simulink model "PhantomX_MK4"  (R2023a)
settings: Solver=FixedStepAuto  StartTime=0.0  StopTime=inf  FixedStep=0.00005  RelTol=1e-3
values from neighbouring files (symbols this model uses):
  angle_offsets_LF_RB = [45, 14.03624347, 60.58440117]    [InitialisationScript.m]    (also in simulation_setup.m)
  angle_offsets_middle = [0, 14.03624347, 60.58440117]    [InitialisationScript.m]    (also in simulation_setup.m)
  angle_offsets_RF_LB = [-45, 14.03624347, 60.58440117]    [InitialisationScript.m]    (also in simulation_setup.m)
  N = 16    [rl_setup.m]
  pid_D = 1    [InitialisationScript.m]    (also in simulation_setup.m)
  pid_filter_N = 100    [InitialisationScript.m]    (also in simulation_setup.m = 1000)
  pid_I = 0.2    [InitialisationScript.m]    (also in simulation_setup.m = 0.1)
  pid_P = 3    [InitialisationScript.m]    (also in simulation_setup.m = 600)
  x_offset = 0.2    [InitialisationScript.m]
  z_offset = -0.14    [InitialisationScript.m]
undefined symbols (not defined in the file or in its folder): LBL_sensory_data, left_side_torques, LFL_sensory_data, LML_sensory_data, RBL_sensory_data, RFL_sensory_data, right_side_torques, RML_sensory_data, X, Y, Z
libraries: sm_lib x30, slpidlib x18, Custom_Library x13, robotmaniplib x6, nesl_utility x3, rllib x1, simulink_extras x1
(part 4 of 4)

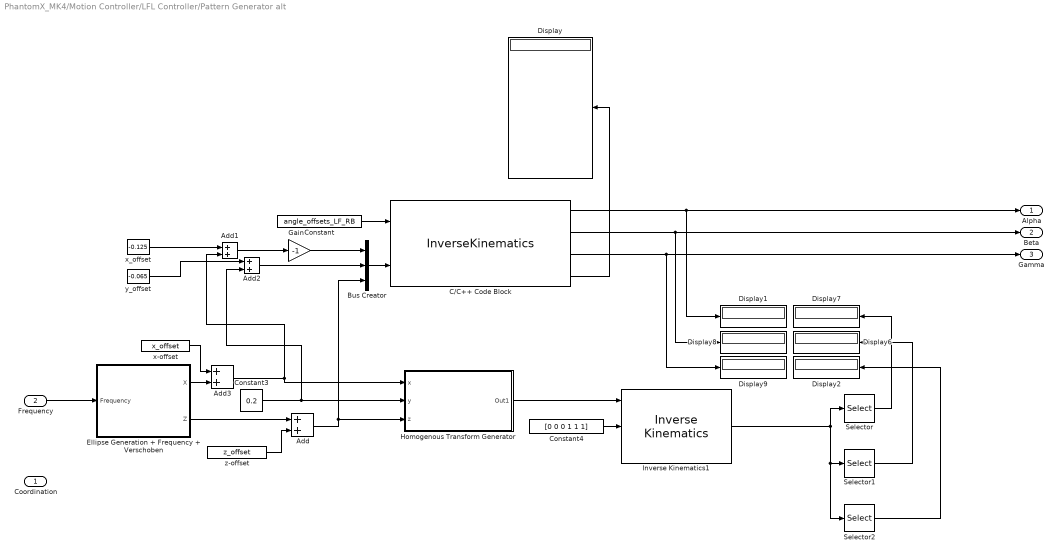
== system PhantomX_MK4/Motion Controller/LFL Controller/Pattern Generator alt ==
  Coordination : Inport
  Frequency : Inport  Port=2
  Add{,1..3} (4 alike) : Sum
  Bus Creator : BusCreator  Inputs=3
  C/C++ Code Block : S-Function  FunctionName=InverseKinematics  SFunctionModules=InverseKinematics_wrapper.c  SFunctionDeploymentMode=off  EnableBusSupport=off  mask(S-Function Builder){}
      mask help: Simulink:masks:SFunctionBuilder_MD
      mask init: same as PhantomX_MK4/Motion Controller/LBL Controller/Pattern Generator alt/C/C++ Code Block
      settings: CopyFcn=set_param(gcbh,'LinkStatus','none')  OpenFcn=sfunctionwizard(gcbh)
      mask Display:
      | plot(val(:,1),val(:,2))
      | disp(sys)
      | port_label('input',1,'angle_offsets')
      | port_label('input',2,'coordinates')
      | port_label('output',1,'alpha')
      | port_label('output',2,'beta')
      | port_label('output',3,'gamma')
      | port_label('output',4,'debug')
  Constant : Constant  Value=angle_offsets_LF_RB
  Constant3 : Constant  Value=0.2
  Constant4 : Constant  Value=[0 0 0 1 1 1]
  Display{,1..2,6..9} (7 alike) : Display
  Ellipse Generation + Frequency + Verschoben : Subsystem
  Gain : Gain  Gain=-1
  Homogenous Transform Generator : Subsystem
  Inverse Kinematics1 : robotmaniplib/Inverse Kinematics  RigidBodyTree=phantomX_mk4  EndEffector=PhantomX_MK4/left_front_foot_link  ShowInfo=off  SolverName=BFGS Gradient Projection  EnforceJointLimits=on  MaxIterations=30  MaxTime=0.01  GradientTolerance=1e-7  SolutionTolerance=1e-6  StepTolerance=1e-14  ErrorChangeTolerance=1e-12  UseErrorDamping=on  DampingBias=0.0025  SimulateUsing=Code generation
  Selector : Selector  IndexMode=Zero-based  InputPortWidth=18  IndexOptions=Starting index (dialog)  Indices=3  OutputSizes=1
  Selector1 : Selector  IndexMode=Zero-based  InputPortWidth=18  IndexOptions=Starting index (dialog)  Indices=4  OutputSizes=1
  Selector2 : Selector  IndexMode=Zero-based  InputPortWidth=18  IndexOptions=Starting index (dialog)  Indices=5  OutputSizes=1
  x-offset : Constant  Value=x_offset
  x_offset : Constant  Value=-0.125
  y_offset : Constant  Value=-0.065
  z-offset : Constant  Value=z_offset
  Alpha : Outport
  Beta : Outport  Port=2
  Gamma : Outport  Port=3
  wires:
  Inverse Kinematics1/1 -> Selector/1, Selector2/1, Selector1/1
  Ellipse Generation + Frequency + Verschoben/2(Z) -> Add/1
  Constant4/1 -> Inverse Kinematics1/2
  Homogenous Transform Generator/1(Out1) -> Inverse Kinematics1/1
  z-offset/1 -> Add/2
  Frequency/1 -> Ellipse Generation + Frequency + Verschoben/1(Frequency)
  C/C++ Code Block/4 -> Display/1
  Ellipse Generation + Frequency + Verschoben/1(X) -> Add3/2
  Add/1 -> Bus Creator/3, Homogenous Transform Generator/3(z)
  Constant3/1 -> Add2/2, Homogenous Transform Generator/2(y)
  C/C++ Code Block/3 -> Display9/1, Gamma/1
  C/C++ Code Block/2 -> Display8/1, Beta/1
  C/C++ Code Block/1 -> Display1/1, Alpha/1
  Selector/1 -> Display7/1
  Selector1/1 -> Display6/1
  Selector2/1 -> Display2/1
  Add2/1 -> Bus Creator/2
  y_offset/1 -> Add2/1
  x_offset/1 -> Add1/1
  Bus Creator/1 -> C/C++ Code Block/2
  Constant/1 -> C/C++ Code Block/1
  Add1/1 -> Gain/1
  Add3/1 -> Add1/2, Homogenous Transform Generator/1(x)
  x-offset/1 -> Add3/1
  Gain/1 -> Bus Creator/1

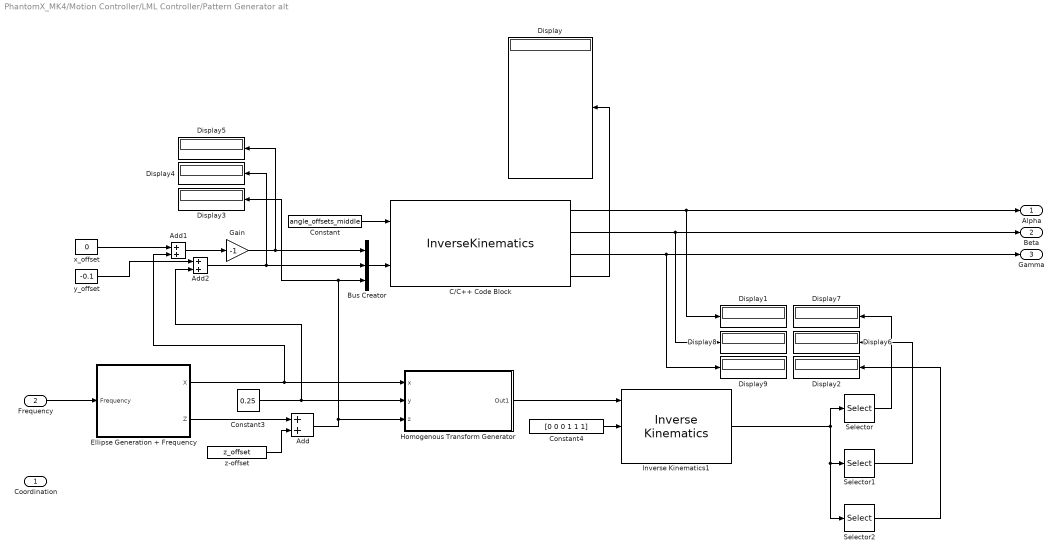
== system PhantomX_MK4/Motion Controller/LML Controller/Pattern Generator alt ==
  Coordination : Inport
  Frequency : Inport  Port=2
  Add : Sum
  Add1 : Sum
  Add2 : Sum
  Bus Creator : BusCreator  Inputs=3
  C/C++ Code Block : S-Function  FunctionName=InverseKinematics  SFunctionModules=InverseKinematics_wrapper.c  SFunctionDeploymentMode=off  EnableBusSupport=off  mask(S-Function Builder){}
      mask help: Simulink:masks:SFunctionBuilder_MD
      mask init: same as PhantomX_MK4/Motion Controller/LBL Controller/Pattern Generator alt/C/C++ Code Block
      settings: CopyFcn=set_param(gcbh,'LinkStatus','none')  OpenFcn=sfunctionwizard(gcbh)
      mask Display:
      | plot(val(:,1),val(:,2))
      | disp(sys)
      | port_label('input',1,'angle_offsets')
      | port_label('input',2,'coordinates')
      | port_label('output',1,'alpha')
      | port_label('output',2,'beta')
      | port_label('output',3,'gamma')
      | port_label('output',4,'debug')
  Constant : Constant  Value=angle_offsets_middle
  Constant3 : Constant  Value=0.25
  Constant4 : Constant  Value=[0 0 0 1 1 1]
  Display{,1..9} (10 alike) : Display
  Ellipse Generation + Frequency : Subsystem
  Gain : Gain  Gain=-1
  Homogenous Transform Generator : Subsystem
  Inverse Kinematics1 : robotmaniplib/Inverse Kinematics  RigidBodyTree=phantomX_mk4  EndEffector=PhantomX_MK4/left_middle_foot_link  ShowInfo=off  SolverName=BFGS Gradient Projection  EnforceJointLimits=on  MaxIterations=30  MaxTime=0.01  GradientTolerance=1e-7  SolutionTolerance=1e-6  StepTolerance=1e-14  ErrorChangeTolerance=1e-12  UseErrorDamping=on  DampingBias=0.0025  SimulateUsing=Code generation
  Selector : Selector  IndexMode=Zero-based  InputPortWidth=18  IndexOptions=Starting index (dialog)  Indices=6  OutputSizes=1
  Selector1 : Selector  IndexMode=Zero-based  InputPortWidth=18  IndexOptions=Starting index (dialog)  Indices=7  OutputSizes=1
  Selector2 : Selector  IndexMode=Zero-based  InputPortWidth=18  IndexOptions=Starting index (dialog)  Indices=8  OutputSizes=1
  x_offset : Constant  Value=0
  y_offset : Constant  Value=-0.1
  z-offset : Constant  Value=z_offset
  Alpha : Outport
  Beta : Outport  Port=2
  Gamma : Outport  Port=3
  wires:
  Inverse Kinematics1/1 -> Selector/1, Selector2/1, Selector1/1
  Ellipse Generation + Frequency/2(Z) -> Add/1
  Constant4/1 -> Inverse Kinematics1/2
  Homogenous Transform Generator/1(Out1) -> Inverse Kinematics1/1
  z-offset/1 -> Add/2
  Frequency/1 -> Ellipse Generation + Frequency/1(Frequency)
  C/C++ Code Block/4 -> Display/1
  Ellipse Generation + Frequency/1(X) -> Add1/2, Homogenous Transform Generator/1(x)
  Add/1 -> Display3/1, Bus Creator/3, Homogenous Transform Generator/3(z)
  Constant3/1 -> Add2/2, Homogenous Transform Generator/2(y)
  C/C++ Code Block/3 -> Display9/1, Gamma/1
  C/C++ Code Block/2 -> Display8/1, Beta/1
  C/C++ Code Block/1 -> Display1/1, Alpha/1
  Selector/1 -> Display7/1
  Selector1/1 -> Display6/1
  Selector2/1 -> Display2/1
  Add2/1 -> Display4/1, Bus Creator/2
  y_offset/1 -> Add2/1
  x_offset/1 -> Add1/1
  Bus Creator/1 -> C/C++ Code Block/2
  Constant/1 -> C/C++ Code Block/1
  Add1/1 -> Gain/1
  Gain/1 -> Display5/1, Bus Creator/1

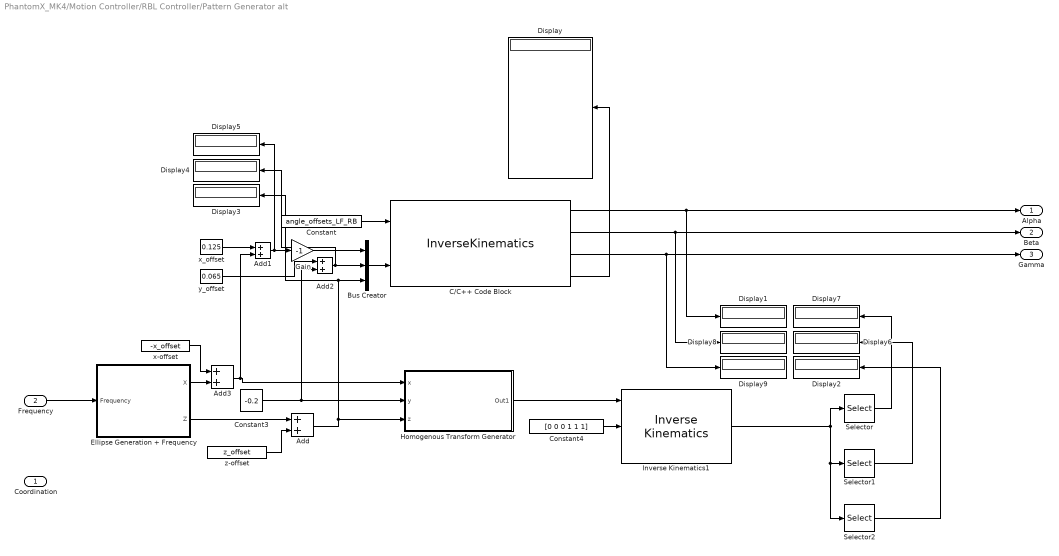
== system PhantomX_MK4/Motion Controller/RBL Controller/Pattern Generator alt ==
  Coordination : Inport
  Frequency : Inport  Port=2
  Add{,1..3} (4 alike) : Sum
  Bus Creator : BusCreator  Inputs=3
  C/C++ Code Block : S-Function  FunctionName=InverseKinematics  SFunctionModules=InverseKinematics_wrapper.c  SFunctionDeploymentMode=off  EnableBusSupport=off  mask(S-Function Builder){}
      mask help: Simulink:masks:SFunctionBuilder_MD
      mask init: same as PhantomX_MK4/Motion Controller/LBL Controller/Pattern Generator alt/C/C++ Code Block
      settings: CopyFcn=set_param(gcbh,'LinkStatus','none')  OpenFcn=sfunctionwizard(gcbh)
      mask Display:
      | plot(val(:,1),val(:,2))
      | disp(sys)
      | port_label('input',1,'angle_offsets')
      | port_label('input',2,'coordinates')
      | port_label('output',1,'alpha')
      | port_label('output',2,'beta')
      | port_label('output',3,'gamma')
      | port_label('output',4,'debug')
  Constant : Constant  Value=angle_offsets_LF_RB
  Constant3 : Constant  Value=-0.2
  Constant4 : Constant  Value=[0 0 0 1 1 1]
  Display{,1..9} (10 alike) : Display
  Ellipse Generation + Frequency : Subsystem
  Gain : Gain  Gain=-1
  Homogenous Transform Generator : Subsystem
  Inverse Kinematics1 : robotmaniplib/Inverse Kinematics  RigidBodyTree=phantomX_mk4  EndEffector=PhantomX_MK4/right_back_foot_link  ShowInfo=off  SolverName=BFGS Gradient Projection  EnforceJointLimits=on  MaxIterations=30  MaxTime=0.01  GradientTolerance=1e-7  SolutionTolerance=1e-6  StepTolerance=1e-14  ErrorChangeTolerance=1e-12  UseErrorDamping=on  DampingBias=0.0025  SimulateUsing=Code generation
  Selector : Selector  IndexMode=Zero-based  InputPortWidth=18  IndexOptions=Starting index (dialog)  Indices=9  OutputSizes=1
  Selector1 : Selector  IndexMode=Zero-based  InputPortWidth=18  IndexOptions=Starting index (dialog)  Indices=10  OutputSizes=1
  Selector2 : Selector  IndexMode=Zero-based  InputPortWidth=18  IndexOptions=Starting index (dialog)  Indices=11  OutputSizes=1
  x-offset : Constant  Value=-x_offset
  x_offset : Constant  Value=0.125
  y_offset : Constant  Value=0.065
  z-offset : Constant  Value=z_offset
  Alpha : Outport
  Beta : Outport  Port=2
  Gamma : Outport  Port=3
  wires:
  Inverse Kinematics1/1 -> Selector/1, Selector2/1, Selector1/1
  Ellipse Generation + Frequency/2(Z) -> Add/1
  Constant4/1 -> Inverse Kinematics1/2
  Homogenous Transform Generator/1(Out1) -> Inverse Kinematics1/1
  z-offset/1 -> Add/2
  Frequency/1 -> Ellipse Generation + Frequency/1(Frequency)
  C/C++ Code Block/4 -> Display/1
  Ellipse Generation + Frequency/1(X) -> Add3/2
  Add/1 -> Display3/1, Bus Creator/3, Homogenous Transform Generator/3(z)
  Constant3/1 -> Add2/2, Homogenous Transform Generator/2(y)
  C/C++ Code Block/3 -> Display9/1, Gamma/1
  C/C++ Code Block/2 -> Display8/1, Beta/1
  C/C++ Code Block/1 -> Display1/1, Alpha/1
  Selector/1 -> Display7/1
  Selector1/1 -> Display6/1
  Selector2/1 -> Display2/1
  Add2/1 -> Display4/1, Bus Creator/2
  y_offset/1 -> Add2/1
  x_offset/1 -> Add1/1
  Bus Creator/1 -> C/C++ Code Block/2
  Constant/1 -> C/C++ Code Block/1
  x-offset/1 -> Add3/1
  Add3/1 -> Add1/2, Homogenous Transform Generator/1(x)
  Add1/1 -> Gain/1, Display5/1
  Gain/1 -> Bus Creator/1

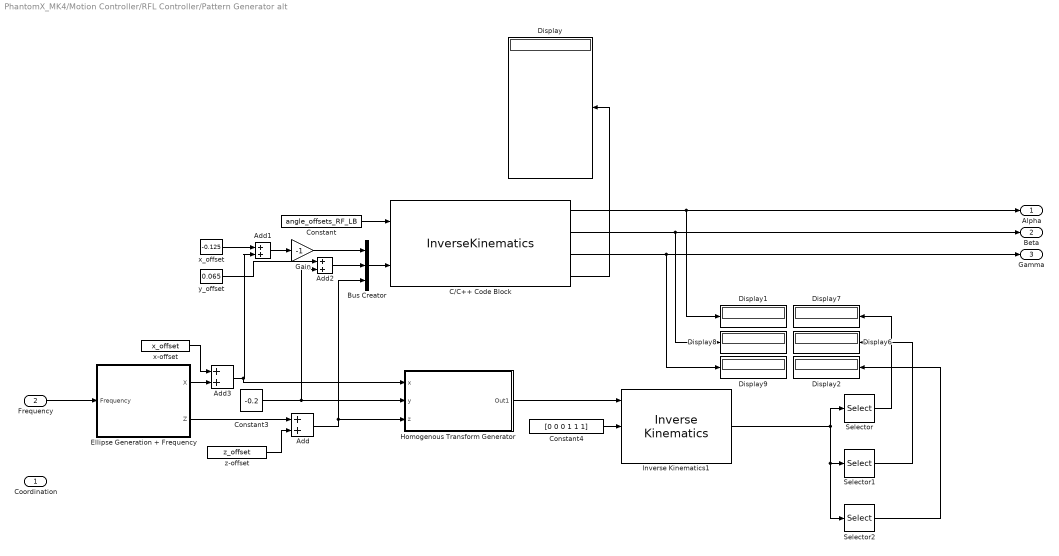
== system PhantomX_MK4/Motion Controller/RFL Controller/Pattern Generator alt ==
  Coordination : Inport
  Frequency : Inport  Port=2
  Add{,1..3} (4 alike) : Sum
  Bus Creator : BusCreator  Inputs=3
  C/C++ Code Block : S-Function  FunctionName=InverseKinematics  SFunctionModules=InverseKinematics_wrapper.c  SFunctionDeploymentMode=off  EnableBusSupport=off  mask(S-Function Builder){}
      mask help: Simulink:masks:SFunctionBuilder_MD
      mask init: same as PhantomX_MK4/Motion Controller/LBL Controller/Pattern Generator alt/C/C++ Code Block
      settings: CopyFcn=set_param(gcbh,'LinkStatus','none')  OpenFcn=sfunctionwizard(gcbh)
      mask Display:
      | plot(val(:,1),val(:,2))
      | disp(sys)
      | port_label('input',1,'angle_offsets')
      | port_label('input',2,'coordinates')
      | port_label('output',1,'alpha')
      | port_label('output',2,'beta')
      | port_label('output',3,'gamma')
      | port_label('output',4,'debug')
  Constant : Constant  Value=angle_offsets_RF_LB
  Constant3 : Constant  Value=-0.2
  Constant4 : Constant  Value=[0 0 0 1 1 1]
  Display{,1..2,6..9} (7 alike) : Display
  Ellipse Generation + Frequency : Subsystem
  Gain : Gain  Gain=-1
  Homogenous Transform Generator : Subsystem
  Inverse Kinematics1 : robotmaniplib/Inverse Kinematics  RigidBodyTree=phantomX_mk4  EndEffector=PhantomX_MK4/right_front_foot_link  ShowInfo=off  SolverName=BFGS Gradient Projection  EnforceJointLimits=on  MaxIterations=30  MaxTime=0.01  GradientTolerance=1e-7  SolutionTolerance=1e-6  StepTolerance=1e-14  ErrorChangeTolerance=1e-12  UseErrorDamping=on  DampingBias=0.0025  SimulateUsing=Code generation
  Selector : Selector  IndexMode=Zero-based  InputPortWidth=18  IndexOptions=Starting index (dialog)  Indices=12  OutputSizes=1
  Selector1 : Selector  IndexMode=Zero-based  InputPortWidth=18  IndexOptions=Starting index (dialog)  Indices=13  OutputSizes=1
  Selector2 : Selector  IndexMode=Zero-based  InputPortWidth=18  IndexOptions=Starting index (dialog)  Indices=14  OutputSizes=1
  x-offset : Constant  Value=x_offset
  x_offset : Constant  Value=-0.125
  y_offset : Constant  Value=0.065
  z-offset : Constant  Value=z_offset
  Alpha : Outport
  Beta : Outport  Port=2
  Gamma : Outport  Port=3
  wires:
  Inverse Kinematics1/1 -> Selector/1, Selector2/1, Selector1/1
  Ellipse Generation + Frequency/2(Z) -> Add/1
  Constant4/1 -> Inverse Kinematics1/2
  Homogenous Transform Generator/1(Out1) -> Inverse Kinematics1/1
  z-offset/1 -> Add/2
  Frequency/1 -> Ellipse Generation + Frequency/1(Frequency)
  C/C++ Code Block/4 -> Display/1
  Ellipse Generation + Frequency/1(X) -> Add3/2
  Add/1 -> Bus Creator/3, Homogenous Transform Generator/3(z)
  Constant3/1 -> Add2/2, Homogenous Transform Generator/2(y)
  C/C++ Code Block/3 -> Display9/1, Gamma/1
  C/C++ Code Block/2 -> Display8/1, Beta/1
  C/C++ Code Block/1 -> Display1/1, Alpha/1
  Selector/1 -> Display7/1
  Selector1/1 -> Display6/1
  Selector2/1 -> Display2/1
  Add2/1 -> Bus Creator/2
  y_offset/1 -> Add2/1
  x_offset/1 -> Add1/1
  Bus Creator/1 -> C/C++ Code Block/2
  Constant/1 -> C/C++ Code Block/1
  x-offset/1 -> Add3/1
  Add1/1 -> Gain/1
  Add3/1 -> Add1/2, Homogenous Transform Generator/1(x)
  Gain/1 -> Bus Creator/1

== system PhantomX_MK4/Motion Controller/RML Controller/Pattern Generator alt ==
  Coordination : Inport
  Frequency : Inport  Port=2
  Add : Sum
  Add1 : Sum
  Add2 : Sum
  Bus Creator : BusCreator  Inputs=3
  C/C++ Code Block : S-Function  FunctionName=InverseKinematics  SFunctionModules=InverseKinematics_wrapper.c  SFunctionDeploymentMode=off  EnableBusSupport=off  mask(S-Function Builder){}
      mask help: Simulink:masks:SFunctionBuilder_MD
      mask init: same as PhantomX_MK4/Motion Controller/LBL Controller/Pattern Generator alt/C/C++ Code Block
      settings: CopyFcn=set_param(gcbh,'LinkStatus','none')  OpenFcn=sfunctionwizard(gcbh)
      mask Display:
      | plot(val(:,1),val(:,2))
      | disp(sys)
      | port_label('input',1,'initial_angles')
      | port_label('input',2,'coordinates')
      | port_label('output',1,'alpha')
      | port_label('output',2,'beta')
      | port_label('output',3,'gamma')
      | port_label('output',4,'debug')
  Constant : Constant  Value=angle_offsets_middle
  Constant3 : Constant  Value=-0.25
  Constant4 : Constant  Value=[0 0 0 1 1 1]
  Display{,1..2,6..9} (7 alike) : Display
  Ellipse Generation + Frequency + Verschoben : Subsystem
  Gain : Gain  Gain=-1
  Homogenous Transform Generator : Subsystem
  Inverse Kinematics1 : robotmaniplib/Inverse Kinematics  RigidBodyTree=phantomX_mk4  EndEffector=PhantomX_MK4/right_middle_foot_link  ShowInfo=off  SolverName=BFGS Gradient Projection  EnforceJointLimits=on  MaxIterations=30  MaxTime=0.01  GradientTolerance=1e-7  SolutionTolerance=1e-6  StepTolerance=1e-14  ErrorChangeTolerance=1e-12  UseErrorDamping=on  DampingBias=0.0025  SimulateUsing=Code generation
  Selector : Selector  IndexMode=Zero-based  InputPortWidth=18  IndexOptions=Starting index (dialog)  Indices=15  OutputSizes=1
  Selector1 : Selector  IndexMode=Zero-based  InputPortWidth=18  IndexOptions=Starting index (dialog)  Indices=16  OutputSizes=1
  Selector2 : Selector  IndexMode=Zero-based  InputPortWidth=18  IndexOptions=Starting index (dialog)  Indices=17  OutputSizes=1
  x_offset : Constant  Value=0
  y_offset : Constant  Value=0.1
  z-offset : Constant  Value=z_offset
  Alpha : Outport
  Beta : Outport  Port=2
  Gamma : Outport  Port=3
  wires:
  Inverse Kinematics1/1 -> Selector/1, Selector2/1, Selector1/1
  Ellipse Generation + Frequency + Verschoben/2(Z) -> Add/1
  Constant4/1 -> Inverse Kinematics1/2
  Homogenous Transform Generator/1(Out1) -> Inverse Kinematics1/1
  z-offset/1 -> Add/2
  Frequency/1 -> Ellipse Generation + Frequency + Verschoben/1(Frequency)
  C/C++ Code Block/4 -> Display/1
  Constant3/1 -> Add2/2, Homogenous Transform Generator/2(y)
  C/C++ Code Block/3 -> Display9/1, Gamma/1
  C/C++ Code Block/2 -> Display8/1, Beta/1
  C/C++ Code Block/1 -> Display1/1, Alpha/1
  Selector/1 -> Display7/1
  Selector1/1 -> Display6/1
  Selector2/1 -> Display2/1
  Add2/1 -> Bus Creator/2
  y_offset/1 -> Add2/1
  x_offset/1 -> Add1/1
  Bus Creator/1 -> C/C++ Code Block/2
  Constant/1 -> C/C++ Code Block/1
  Add1/1 -> Gain/1
  Ellipse Generation + Frequency + Verschoben/1(X) -> Add1/2, Homogenous Transform Generator/1(x)
  Add/1 -> Bus Creator/3, Homogenous Transform Generator/3(z)
  Gain/1 -> Bus Creator/1

== system PhantomX_MK4/Physical Robot Model/PhantomX Body/PhantomX_MK4_base_bottom_link ==
  Inertia : sm_lib/Body Elements/Inertia  InertiaType=Custom  Mass=800  MassUnits=g  CenterOfMass=[0, 0, 0]  CenterOfMassUnits=m  MomentsOfInertia=[0, 0, 0]  MomentsOfInertiaUnits=kg*m^2  ProductsOfInertia=[0, 0, 0]  ProductsOfInertiaUnits=kg*m^2  GraphicType=None  MarkerShape=Inertia  MarkerSize=20  GraphicVisPropType=SimpleVisualProperties  GraphicDiffuseColor=[0.5 0.5 0.5]  GraphicSpecularColor=[0.5 0.5 0.5 1.0]  GraphicAmbientColor=[0.15 0.15 0.15 1.0]  GraphicEmissiveColor=[0.0 0.0 0.0 1.0]  GraphicShininess=75  GraphicOpacity=1.0
  InertiaOriginTransform : sm_lib/Frames and Transforms/Rigid Transform  TranslationMethod=Cartesian  TranslationStandardOffset=0  TranslationStandardOffsetUnits=m  TranslationStandardAxis=+Z  TranslationCartesianOffset=[0, 0, 0]  TranslationCartesianOffsetUnits=m  TranslationROffset=0  TranslationROffsetUnits=m  TranslationZOffset=0  TranslationZOffsetUnits=m  TranslationThetaOffset=0  TranslationThetaOffsetUnits=deg  RotationMethod=RotationSequence  RotationAngleUnits=deg  RotationStandardAxis=+Z  RotationAngle=0.0  RotationArbitraryAxis=[0 0 1]  FollAlignAxisA=+X  BaseAlignAxisA=+Y  FollAlignAxisB=+Y  BaseAlignAxisB=+Z  RotationSequenceAxes=BaseAxes  RotationSequence=XYZ  RotationSequenceAngles=[0, 0, 0]  RotationSequenceAnglesUnits=rad  RotationMatrix=[1 0 0; 0 1 0; 0 0 1]  Quaternion=[1 0 0 0]
  ReferenceFrame : sm_lib/Frames and Transforms/Reference Frame
  F : PMIOPort  Side=Left
  connections:
  Inertia/RConn1 -- InertiaOriginTransform/RConn1
  InertiaOriginTransform/LConn1 -- ReferenceFrame/RConn1 -- F/RConn1

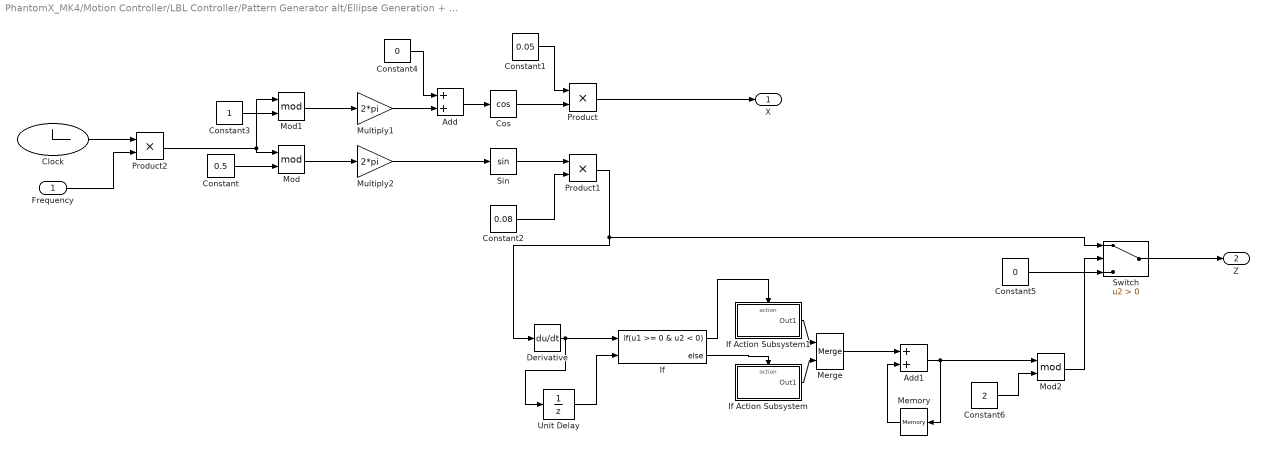
== system PhantomX_MK4/Motion Controller/LBL Controller/Pattern Generator alt/Ellipse Generation + Frequency + Verschoben ==
  Frequency : Inport
  Add : Sum
  Add1 : Sum
  Clock : Clock
  Constant : Constant  Value=0.5
  Constant1 : Constant  Value=0.05
  Constant2 : Constant  Value=0.08
  Constant3 : Constant
  Constant4 : Constant  Value=0
  Constant5 : Constant  Value=0
  Constant6 : Constant  Value=2
  Cos : Trigonometry  Operator=cos
  Derivative : Derivative
  If : If  NumInputs=2  IfExpression=u1 >= 0 & u2 < 0
  If Action Subsystem : Subsystem  TreatAsAtomicUnit=on
  If Action Subsystem1 : Subsystem  TreatAsAtomicUnit=on
  Memory : Memory
  Merge : Merge
  Mod : Math  Operator=mod
  Mod1 : Math  Operator=mod
  Mod2 : Math  Operator=mod
  Multiply1 : Gain  Gain=2*pi
  Multiply2 : Gain  Gain=2*pi
  Product : Product
  Product1 : Product
  Product2 : Product
  Sin : Trigonometry
  Switch : Switch  Criteria=u2 > Threshold  SaturateOnIntegerOverflow=off  InputSameDT=off
  Unit Delay : UnitDelay  SampleTime=-1  HasFrameUpgradeWarning=on
  X : Outport
  Z : Outport  Port=2
  wires:
  Constant/1 -> Mod/2
  Mod/1 -> Multiply2/1
  Sin/1 -> Product1/1
  Cos/1 -> Product/2
  Constant1/1 -> Product/1
  Constant2/1 -> Product1/2
  Product1/1 -> Switch/1, Derivative/1
  Product/1 -> X/1
  Mod1/1 -> Multiply1/1
  Constant3/1 -> Mod1/2
  Add/1 -> Cos/1
  Constant4/1 -> Add/1
  Add1/1 -> Mod2/1, Memory/1
  Memory/1 -> Add1/2
  If/2 -> If Action Subsystem/Action
  If/1 -> If Action Subsystem1/Action
  If Action Subsystem/1(Out1) -> Merge/2
  If Action Subsystem1/1(Out1) -> Merge/1
  Merge/1 -> Add1/1
  Switch/1 -> Z/1
  Constant5/1 -> Switch/3
  Constant6/1 -> Mod2/2
  Mod2/1 -> Switch/2
  Multiply2/1 -> Sin/1
  Frequency/1 -> Product2/2
  Multiply1/1 -> Add/2
  Clock/1 -> Product2/1
  Product2/1 -> Mod1/1, Mod/1
  Derivative/1 -> Unit Delay/1, If/1
  Unit Delay/1 -> If/2

== system PhantomX_MK4/Motion Controller/LBL Controller/Pattern Generator alt/Homogenous Transform Generator ==
  x : Inport
  y : Inport  Port=2
  z : Inport  Port=3
  Constant3 : Constant  Value=[-1 0 0; 0 -1 0; 0 0 1; 0 0 0]
  Constant5 : Constant
  Matrix Concatenate : Concatenate  Mode=Multidimensional array  ConcatenateDimension=2
  Vector Concatenate : Concatenate  NumInputs=4
  Out1 : Outport
  wires:
  z/1 -> Vector Concatenate/3
  Vector Concatenate/1 -> Matrix Concatenate/2
  Constant3/1 -> Matrix Concatenate/1
  Constant5/1 -> Vector Concatenate/4
  x/1 -> Vector Concatenate/1
  Matrix Concatenate/1 -> Out1/1
  y/1 -> Vector Concatenate/2

== system PhantomX_MK4/Motion Controller/LFL Controller/Pattern Generator alt/Ellipse Generation + Frequency + Verschoben ==
  Frequency : Inport
  Add : Sum
  Add1 : Sum
  Clock : Clock
  Constant : Constant  Value=0.5
  Constant1 : Constant  Value=0.05
  Constant2 : Constant  Value=0.08
  Constant3 : Constant
  Constant4 : Constant  Value=0
  Constant5 : Constant  Value=0
  Constant6 : Constant  Value=2
  Cos : Trigonometry  Operator=cos
  Derivative : Derivative
  If : If  NumInputs=2  IfExpression=u1 >= 0 & u2 < 0
  If Action Subsystem : Subsystem  TreatAsAtomicUnit=on
  If Action Subsystem1 : Subsystem  TreatAsAtomicUnit=on
  Memory : Memory
  Merge : Merge
  Mod : Math  Operator=mod
  Mod1 : Math  Operator=mod
  Mod2 : Math  Operator=mod
  Multiply1 : Gain  Gain=2*pi
  Multiply2 : Gain  Gain=2*pi
  Product : Product
  Product1 : Product
  Product2 : Product
  Sin : Trigonometry
  Switch : Switch  Criteria=u2 > Threshold  SaturateOnIntegerOverflow=off  InputSameDT=off
  Unit Delay : UnitDelay  SampleTime=-1  HasFrameUpgradeWarning=on
  X : Outport
  Z : Outport  Port=2
  wires:
  Constant/1 -> Mod/2
  Mod/1 -> Multiply2/1
  Sin/1 -> Product1/1
  Cos/1 -> Product/2
  Constant1/1 -> Product/1
  Constant2/1 -> Product1/2
  Product1/1 -> Switch/1, Derivative/1
  Product/1 -> X/1
  Mod1/1 -> Multiply1/1
  Constant3/1 -> Mod1/2
  Add/1 -> Cos/1
  Constant4/1 -> Add/1
  Add1/1 -> Mod2/1, Memory/1
  Memory/1 -> Add1/2
  If/2 -> If Action Subsystem/Action
  If/1 -> If Action Subsystem1/Action
  If Action Subsystem/1(Out1) -> Merge/2
  If Action Subsystem1/1(Out1) -> Merge/1
  Merge/1 -> Add1/1
  Switch/1 -> Z/1
  Constant5/1 -> Switch/3
  Constant6/1 -> Mod2/2
  Mod2/1 -> Switch/2
  Multiply2/1 -> Sin/1
  Frequency/1 -> Product2/2
  Multiply1/1 -> Add/2
  Clock/1 -> Product2/1
  Product2/1 -> Mod1/1, Mod/1
  Derivative/1 -> Unit Delay/1, If/1
  Unit Delay/1 -> If/2

== system PhantomX_MK4/Motion Controller/LFL Controller/Pattern Generator alt/Homogenous Transform Generator ==
  x : Inport
  y : Inport  Port=2
  z : Inport  Port=3
  Constant3 : Constant  Value=[-1 0 0; 0 -1 0; 0 0 1; 0 0 0]
  Constant5 : Constant
  Matrix Concatenate : Concatenate  Mode=Multidimensional array  ConcatenateDimension=2
  Vector Concatenate : Concatenate  NumInputs=4
  Out1 : Outport
  wires:
  z/1 -> Vector Concatenate/3
  Vector Concatenate/1 -> Matrix Concatenate/2
  Constant3/1 -> Matrix Concatenate/1
  Constant5/1 -> Vector Concatenate/4
  x/1 -> Vector Concatenate/1
  Matrix Concatenate/1 -> Out1/1
  y/1 -> Vector Concatenate/2

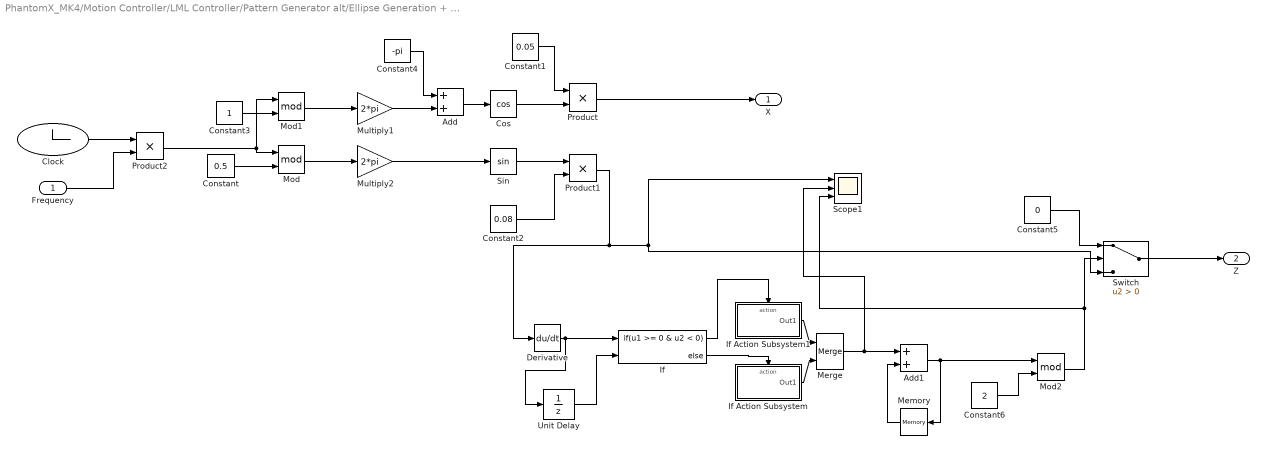
== system PhantomX_MK4/Motion Controller/LML Controller/Pattern Generator alt/Ellipse Generation + Frequency ==
  Frequency : Inport
  Add : Sum
  Add1 : Sum
  Clock : Clock
  Constant : Constant  Value=0.5
  Constant1 : Constant  Value=0.05
  Constant2 : Constant  Value=0.08
  Constant3 : Constant
  Constant4 : Constant  Value=-pi
  Constant5 : Constant  Value=0
  Constant6 : Constant  Value=2
  Cos : Trigonometry  Operator=cos
  Derivative : Derivative
  If : If  NumInputs=2  IfExpression=u1 >= 0 & u2 < 0
  If Action Subsystem : Subsystem  TreatAsAtomicUnit=on
  If Action Subsystem1 : Subsystem  TreatAsAtomicUnit=on
  Memory : Memory
  Merge : Merge
  Mod : Math  Operator=mod
  Mod1 : Math  Operator=mod
  Mod2 : Math  Operator=mod
  Multiply1 : Gain  Gain=2*pi
  Multiply2 : Gain  Gain=2*pi
  Product : Product
  Product1 : Product
  Product2 : Product
  Scope1 : Scope  NumInputPorts=3
  Sin : Trigonometry
  Switch : Switch  Criteria=u2 > Threshold  SaturateOnIntegerOverflow=off  InputSameDT=off
  Unit Delay : UnitDelay  SampleTime=-1  HasFrameUpgradeWarning=on
  X : Outport
  Z : Outport  Port=2
  wires:
  Constant/1 -> Mod/2
  Mod/1 -> Multiply2/1
  Sin/1 -> Product1/1
  Cos/1 -> Product/2
  Constant1/1 -> Product/1
  Constant2/1 -> Product1/2
  Product1/1 -> Derivative/1, Switch/3, Scope1/1
  Product/1 -> X/1
  Mod1/1 -> Multiply1/1
  Constant3/1 -> Mod1/2
  Add/1 -> Cos/1
  Constant4/1 -> Add/1
  Add1/1 -> Mod2/1, Memory/1
  Memory/1 -> Add1/2
  If/2 -> If Action Subsystem/Action
  If/1 -> If Action Subsystem1/Action
  If Action Subsystem/1(Out1) -> Merge/2
  If Action Subsystem1/1(Out1) -> Merge/1
  Switch/1 -> Z/1
  Constant5/1 -> Switch/1
  Constant6/1 -> Mod2/2
  Multiply2/1 -> Sin/1
  Frequency/1 -> Product2/2
  Multiply1/1 -> Add/2
  Clock/1 -> Product2/1
  Product2/1 -> Mod1/1, Mod/1
  Derivative/1 -> Unit Delay/1, If/1
  Unit Delay/1 -> If/2
  Mod2/1 -> Scope1/3, Switch/2
  Merge/1 -> Scope1/2, Add1/1

== system PhantomX_MK4/Motion Controller/LML Controller/Pattern Generator alt/Homogenous Transform Generator ==
  x : Inport
  y : Inport  Port=2
  z : Inport  Port=3
  Constant3 : Constant  Value=[-1 0 0; 0 -1 0; 0 0 1; 0 0 0]
  Constant5 : Constant
  Matrix Concatenate : Concatenate  Mode=Multidimensional array  ConcatenateDimension=2
  Vector Concatenate : Concatenate  NumInputs=4
  Out1 : Outport
  wires:
  z/1 -> Vector Concatenate/3
  Vector Concatenate/1 -> Matrix Concatenate/2
  Constant3/1 -> Matrix Concatenate/1
  Constant5/1 -> Vector Concatenate/4
  x/1 -> Vector Concatenate/1
  Matrix Concatenate/1 -> Out1/1
  y/1 -> Vector Concatenate/2

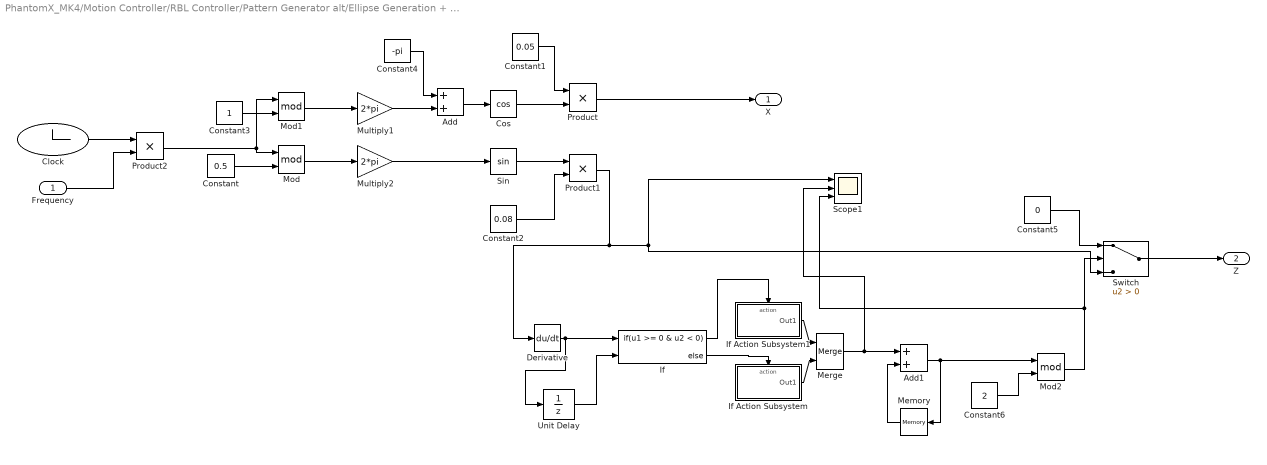
== system PhantomX_MK4/Motion Controller/RBL Controller/Pattern Generator alt/Ellipse Generation + Frequency ==
  Frequency : Inport
  Add : Sum
  Add1 : Sum
  Clock : Clock
  Constant : Constant  Value=0.5
  Constant1 : Constant  Value=0.05
  Constant2 : Constant  Value=0.08
  Constant3 : Constant
  Constant4 : Constant  Value=-pi
  Constant5 : Constant  Value=0
  Constant6 : Constant  Value=2
  Cos : Trigonometry  Operator=cos
  Derivative : Derivative
  If : If  NumInputs=2  IfExpression=u1 >= 0 & u2 < 0
  If Action Subsystem : Subsystem  TreatAsAtomicUnit=on
  If Action Subsystem1 : Subsystem  TreatAsAtomicUnit=on
  Memory : Memory
  Merge : Merge
  Mod : Math  Operator=mod
  Mod1 : Math  Operator=mod
  Mod2 : Math  Operator=mod
  Multiply1 : Gain  Gain=2*pi
  Multiply2 : Gain  Gain=2*pi
  Product : Product
  Product1 : Product
  Product2 : Product
  Scope1 : Scope  NumInputPorts=3
  Sin : Trigonometry
  Switch : Switch  Criteria=u2 > Threshold  SaturateOnIntegerOverflow=off  InputSameDT=off
  Unit Delay : UnitDelay  SampleTime=-1  HasFrameUpgradeWarning=on
  X : Outport
  Z : Outport  Port=2
  wires:
  Constant/1 -> Mod/2
  Mod/1 -> Multiply2/1
  Sin/1 -> Product1/1
  Cos/1 -> Product/2
  Constant1/1 -> Product/1
  Constant2/1 -> Product1/2
  Product1/1 -> Derivative/1, Switch/3, Scope1/1
  Product/1 -> X/1
  Mod1/1 -> Multiply1/1
  Constant3/1 -> Mod1/2
  Add/1 -> Cos/1
  Constant4/1 -> Add/1
  Add1/1 -> Mod2/1, Memory/1
  Memory/1 -> Add1/2
  If/2 -> If Action Subsystem/Action
  If/1 -> If Action Subsystem1/Action
  If Action Subsystem/1(Out1) -> Merge/2
  If Action Subsystem1/1(Out1) -> Merge/1
  Switch/1 -> Z/1
  Constant5/1 -> Switch/1
  Constant6/1 -> Mod2/2
  Multiply2/1 -> Sin/1
  Frequency/1 -> Product2/2
  Multiply1/1 -> Add/2
  Clock/1 -> Product2/1
  Product2/1 -> Mod1/1, Mod/1
  Derivative/1 -> Unit Delay/1, If/1
  Unit Delay/1 -> If/2
  Mod2/1 -> Scope1/3, Switch/2
  Merge/1 -> Scope1/2, Add1/1

== system PhantomX_MK4/Motion Controller/RBL Controller/Pattern Generator alt/Homogenous Transform Generator ==
  x : Inport
  y : Inport  Port=2
  z : Inport  Port=3
  Constant3 : Constant  Value=[-1 0 0; 0 -1 0; 0 0 1; 0 0 0]
  Constant5 : Constant
  Matrix Concatenate : Concatenate  Mode=Multidimensional array  ConcatenateDimension=2
  Vector Concatenate : Concatenate  NumInputs=4
  Out1 : Outport
  wires:
  z/1 -> Vector Concatenate/3
  Vector Concatenate/1 -> Matrix Concatenate/2
  Constant3/1 -> Matrix Concatenate/1
  Constant5/1 -> Vector Concatenate/4
  x/1 -> Vector Concatenate/1
  Matrix Concatenate/1 -> Out1/1
  y/1 -> Vector Concatenate/2

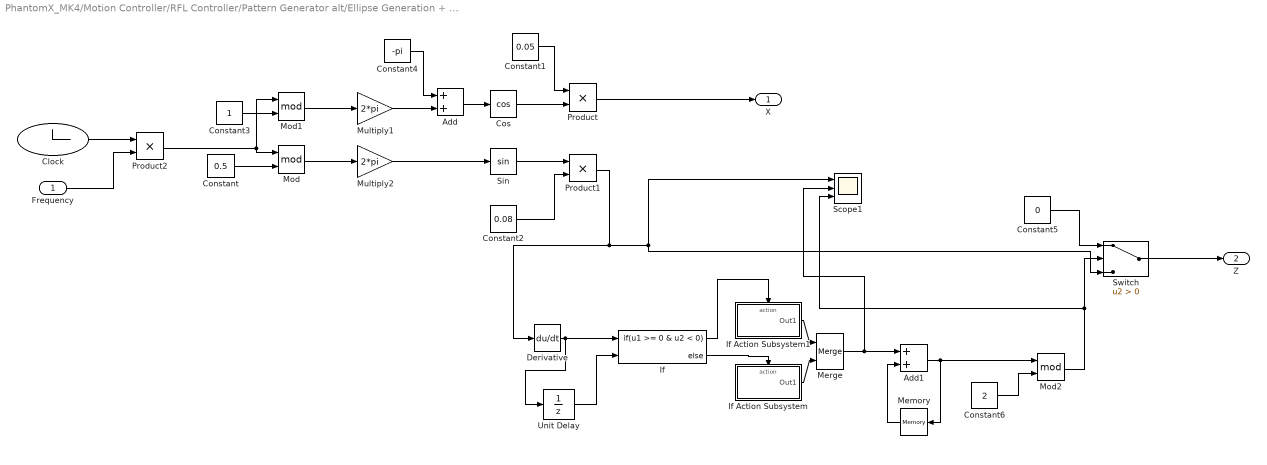
== system PhantomX_MK4/Motion Controller/RFL Controller/Pattern Generator alt/Ellipse Generation + Frequency ==
  Frequency : Inport
  Add : Sum
  Add1 : Sum
  Clock : Clock
  Constant : Constant  Value=0.5
  Constant1 : Constant  Value=0.05
  Constant2 : Constant  Value=0.08
  Constant3 : Constant
  Constant4 : Constant  Value=-pi
  Constant5 : Constant  Value=0
  Constant6 : Constant  Value=2
  Cos : Trigonometry  Operator=cos
  Derivative : Derivative
  If : If  NumInputs=2  IfExpression=u1 >= 0 & u2 < 0
  If Action Subsystem : Subsystem  TreatAsAtomicUnit=on
  If Action Subsystem1 : Subsystem  TreatAsAtomicUnit=on
  Memory : Memory
  Merge : Merge
  Mod : Math  Operator=mod
  Mod1 : Math  Operator=mod
  Mod2 : Math  Operator=mod
  Multiply1 : Gain  Gain=2*pi
  Multiply2 : Gain  Gain=2*pi
  Product : Product
  Product1 : Product
  Product2 : Product
  Scope1 : Scope  NumInputPorts=3
  Sin : Trigonometry
  Switch : Switch  Criteria=u2 > Threshold  SaturateOnIntegerOverflow=off  InputSameDT=off
  Unit Delay : UnitDelay  SampleTime=-1  HasFrameUpgradeWarning=on
  X : Outport
  Z : Outport  Port=2
  wires:
  Constant/1 -> Mod/2
  Mod/1 -> Multiply2/1
  Sin/1 -> Product1/1
  Cos/1 -> Product/2
  Constant1/1 -> Product/1
  Constant2/1 -> Product1/2
  Product1/1 -> Derivative/1, Switch/3, Scope1/1
  Product/1 -> X/1
  Mod1/1 -> Multiply1/1
  Constant3/1 -> Mod1/2
  Add/1 -> Cos/1
  Constant4/1 -> Add/1
  Add1/1 -> Mod2/1, Memory/1
  Memory/1 -> Add1/2
  If/2 -> If Action Subsystem/Action
  If/1 -> If Action Subsystem1/Action
  If Action Subsystem/1(Out1) -> Merge/2
  If Action Subsystem1/1(Out1) -> Merge/1
  Switch/1 -> Z/1
  Constant5/1 -> Switch/1
  Constant6/1 -> Mod2/2
  Multiply2/1 -> Sin/1
  Frequency/1 -> Product2/2
  Multiply1/1 -> Add/2
  Clock/1 -> Product2/1
  Product2/1 -> Mod1/1, Mod/1
  Derivative/1 -> Unit Delay/1, If/1
  Unit Delay/1 -> If/2
  Mod2/1 -> Scope1/3, Switch/2
  Merge/1 -> Scope1/2, Add1/1

== system PhantomX_MK4/Motion Controller/RFL Controller/Pattern Generator alt/Homogenous Transform Generator ==
  x : Inport
  y : Inport  Port=2
  z : Inport  Port=3
  Constant3 : Constant  Value=[-1 0 0; 0 -1 0; 0 0 1; 0 0 0]
  Constant5 : Constant
  Matrix Concatenate : Concatenate  Mode=Multidimensional array  ConcatenateDimension=2
  Vector Concatenate : Concatenate  NumInputs=4
  Out1 : Outport
  wires:
  z/1 -> Vector Concatenate/3
  Vector Concatenate/1 -> Matrix Concatenate/2
  Constant3/1 -> Matrix Concatenate/1
  Constant5/1 -> Vector Concatenate/4
  x/1 -> Vector Concatenate/1
  Matrix Concatenate/1 -> Out1/1
  y/1 -> Vector Concatenate/2

== system PhantomX_MK4/Motion Controller/RML Controller/Pattern Generator alt/Ellipse Generation + Frequency + Verschoben ==
  Frequency : Inport
  Add : Sum
  Add1 : Sum
  Clock : Clock
  Constant : Constant  Value=0.5
  Constant1 : Constant  Value=0.05
  Constant2 : Constant  Value=0.08
  Constant3 : Constant
  Constant4 : Constant  Value=0
  Constant5 : Constant  Value=0
  Constant6 : Constant  Value=2
  Cos : Trigonometry  Operator=cos
  Derivative : Derivative
  If : If  NumInputs=2  IfExpression=u1 >= 0 & u2 < 0
  If Action Subsystem : Subsystem  TreatAsAtomicUnit=on
  If Action Subsystem1 : Subsystem  TreatAsAtomicUnit=on
  Memory : Memory
  Merge : Merge
  Mod : Math  Operator=mod
  Mod1 : Math  Operator=mod
  Mod2 : Math  Operator=mod
  Multiply1 : Gain  Gain=2*pi
  Multiply2 : Gain  Gain=2*pi
  Product : Product
  Product1 : Product
  Product2 : Product
  Sin : Trigonometry
  Switch : Switch  Criteria=u2 > Threshold  SaturateOnIntegerOverflow=off  InputSameDT=off
  Unit Delay : UnitDelay  SampleTime=-1  HasFrameUpgradeWarning=on
  X : Outport
  Z : Outport  Port=2
  wires:
  Constant/1 -> Mod/2
  Mod/1 -> Multiply2/1
  Sin/1 -> Product1/1
  Cos/1 -> Product/2
  Constant1/1 -> Product/1
  Constant2/1 -> Product1/2
  Product1/1 -> Switch/1, Derivative/1
  Product/1 -> X/1
  Mod1/1 -> Multiply1/1
  Constant3/1 -> Mod1/2
  Add/1 -> Cos/1
  Constant4/1 -> Add/1
  Add1/1 -> Mod2/1, Memory/1
  Memory/1 -> Add1/2
  If/2 -> If Action Subsystem/Action
  If/1 -> If Action Subsystem1/Action
  If Action Subsystem/1(Out1) -> Merge/2
  If Action Subsystem1/1(Out1) -> Merge/1
  Merge/1 -> Add1/1
  Switch/1 -> Z/1
  Constant5/1 -> Switch/3
  Constant6/1 -> Mod2/2
  Mod2/1 -> Switch/2
  Multiply2/1 -> Sin/1
  Frequency/1 -> Product2/2
  Multiply1/1 -> Add/2
  Clock/1 -> Product2/1
  Product2/1 -> Mod1/1, Mod/1
  Derivative/1 -> Unit Delay/1, If/1
  Unit Delay/1 -> If/2

== system PhantomX_MK4/Motion Controller/RML Controller/Pattern Generator alt/Homogenous Transform Generator ==
  x : Inport
  y : Inport  Port=2
  z : Inport  Port=3
  Constant3 : Constant  Value=[-1 0 0; 0 -1 0; 0 0 1; 0 0 0]
  Constant5 : Constant
  Matrix Concatenate : Concatenate  Mode=Multidimensional array  ConcatenateDimension=2
  Vector Concatenate : Concatenate  NumInputs=4
  Out1 : Outport
  wires:
  z/1 -> Vector Concatenate/3
  Vector Concatenate/1 -> Matrix Concatenate/2
  Constant3/1 -> Matrix Concatenate/1
  Constant5/1 -> Vector Concatenate/4
  x/1 -> Vector Concatenate/1
  Matrix Concatenate/1 -> Out1/1
  y/1 -> Vector Concatenate/2

== system PhantomX_MK4/Motion Controller/LBL Controller/Pattern Generator alt/Ellipse Generation + Frequency + Verschoben/If Action Subsystem ==
  Action Port : ActionPort
  Constant : Constant  Value=0
  Out1 : Outport
  wires:
  Constant/1 -> Out1/1

== system PhantomX_MK4/Motion Controller/LBL Controller/Pattern Generator alt/Ellipse Generation + Frequency + Verschoben/If Action Subsystem1 ==
  Action Port : ActionPort
  Constant : Constant
  Out1 : Outport
  wires:
  Constant/1 -> Out1/1

== system PhantomX_MK4/Motion Controller/LFL Controller/Pattern Generator alt/Ellipse Generation + Frequency + Verschoben/If Action Subsystem ==
  Action Port : ActionPort
  Constant : Constant  Value=0
  Out1 : Outport
  wires:
  Constant/1 -> Out1/1

== system PhantomX_MK4/Motion Controller/LFL Controller/Pattern Generator alt/Ellipse Generation + Frequency + Verschoben/If Action Subsystem1 ==
  Action Port : ActionPort
  Constant : Constant
  Out1 : Outport
  wires:
  Constant/1 -> Out1/1

== system PhantomX_MK4/Motion Controller/LML Controller/Pattern Generator alt/Ellipse Generation + Frequency/If Action Subsystem ==
  Action Port : ActionPort
  Constant : Constant  Value=0
  Out1 : Outport
  wires:
  Constant/1 -> Out1/1

== system PhantomX_MK4/Motion Controller/LML Controller/Pattern Generator alt/Ellipse Generation + Frequency/If Action Subsystem1 ==
  Action Port : ActionPort
  Constant : Constant
  Out1 : Outport
  wires:
  Constant/1 -> Out1/1

== system PhantomX_MK4/Motion Controller/RBL Controller/Pattern Generator alt/Ellipse Generation + Frequency/If Action Subsystem ==
  Action Port : ActionPort
  Constant : Constant  Value=0
  Out1 : Outport
  wires:
  Constant/1 -> Out1/1

== system PhantomX_MK4/Motion Controller/RBL Controller/Pattern Generator alt/Ellipse Generation + Frequency/If Action Subsystem1 ==
  Action Port : ActionPort
  Constant : Constant
  Out1 : Outport
  wires:
  Constant/1 -> Out1/1

== system PhantomX_MK4/Motion Controller/RFL Controller/Pattern Generator alt/Ellipse Generation + Frequency/If Action Subsystem ==
  Action Port : ActionPort  ActionPortLabel=else
  Constant : Constant  Value=0
  Out1 : Outport
  wires:
  Constant/1 -> Out1/1

== system PhantomX_MK4/Motion Controller/RFL Controller/Pattern Generator alt/Ellipse Generation + Frequency/If Action Subsystem1 ==
  Action Port : ActionPort  ActionPortLabel=if(u1 >= 0 & u2 < 0)
  Constant : Constant
  Out1 : Outport
  wires:
  Constant/1 -> Out1/1

== system PhantomX_MK4/Motion Controller/RML Controller/Pattern Generator alt/Ellipse Generation + Frequency + Verschoben/If Action Subsystem ==
  Action Port : ActionPort
  Constant : Constant  Value=0
  Out1 : Outport
  wires:
  Constant/1 -> Out1/1

== system PhantomX_MK4/Motion Controller/RML Controller/Pattern Generator alt/Ellipse Generation + Frequency + Verschoben/If Action Subsystem1 ==
  Action Port : ActionPort
  Constant : Constant
  Out1 : Outport
  wires:
  Constant/1 -> Out1/1
